simulink model "TP"  (Simulink 8.2)
settings: Solver=ode3  StartTime=0.0  StopTime=50  FixedStep=0.001  RelTol=1e-3
undefined symbols (not defined in the file): D, K, T, w
settings Model: Creator=daniw  LastModifiedBy=daniw
settings DataIOCC: LimitDataPoints=off  SignalLoggingSaveFormat=Dataset
settings OptimizationCC: ExpressionDepthLimit=128
settings DebuggingCC: FcnCallInpInsideContextMsg=EnableAllAsError  StateNameClashWarn=none
settings GRTTargetCC: CombineOutputUpdateFcns=on  GRTInterface=off

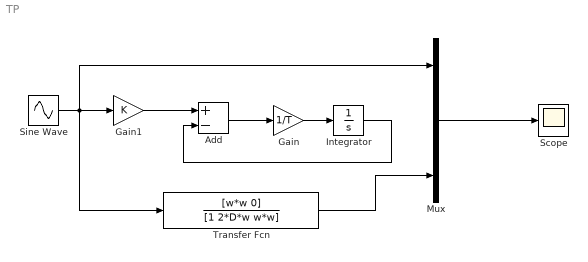
== system TP ==
  Add : Sum  Inputs=+-
  Gain : Gain  Gain=1/T
  Gain1 : Gain  Gain=K
  Integrator : Integrator  InitialCondition=1
  Mux : Mux  Inputs=3
  Scope : Scope
  Sine Wave : Sin  Frequency=4  SampleTime=0
  Transfer Fcn : TransferFcn  Numerator=[w*w 0]  Denominator=[1 2*D*w w*w]
  wires:
  Sine Wave/1 -> Transfer Fcn/1, Mux/1, Gain1/1
  Gain1/1 -> Add/1
  Add/1 -> Gain/1
  Gain/1 -> Integrator/1
  Integrator/1 -> Add/2
  Transfer Fcn/1 -> Mux/3
  Mux/1 -> Scope/1
